simulink subsystem "control_filter"  (R2022b)
settings: Solver=VariableStepAuto  StartTime=0.0  StopTime=10.0  RelTol=1e-3
libraries: simulink x4, SG_library x1, hdlsllib x1
settings Model: Creator=mavolery  LastModifiedBy=mavolery

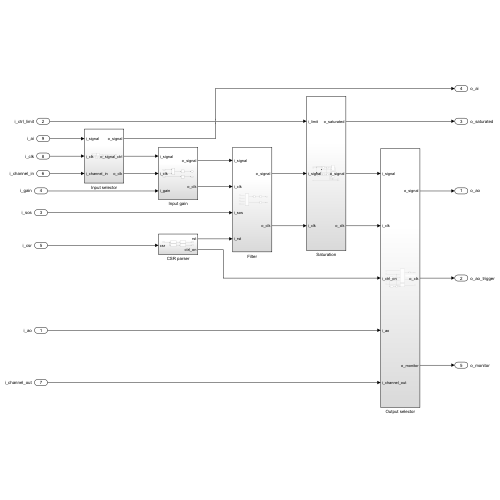
[thumbnail: Simulink's stored preview of the top-level diagram]
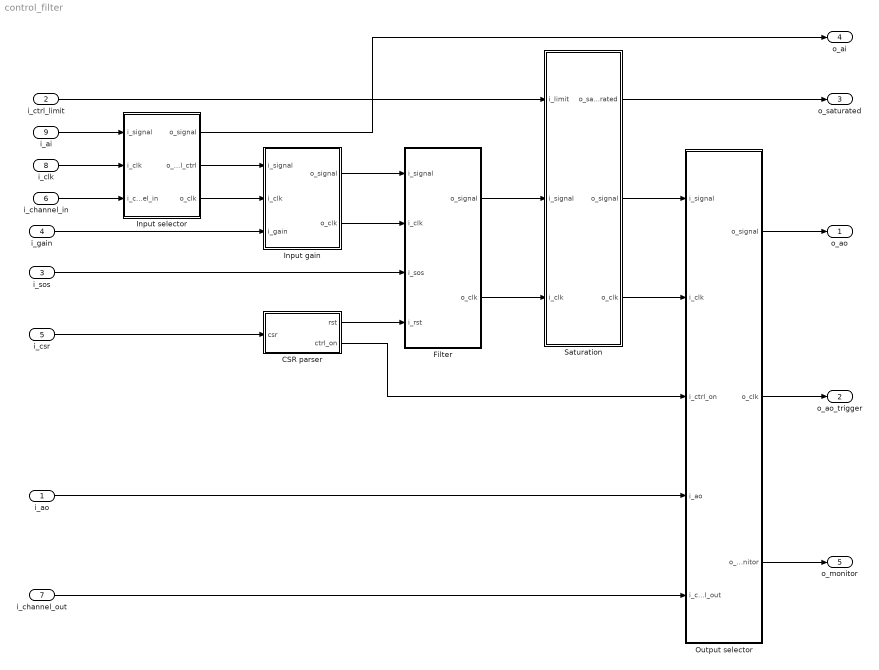
== system control_filter ==
  i_ao : Inport  OutDataTypeStr=fixdt(1,16,15)
  i_ctrl_limit : Inport  Port=2  OutDataTypeStr=fixdt(1,16,15)
  i_sos : Inport  Port=3  OutDataTypeStr=fixdt(1,32,26)
  i_gain : Inport  Port=4  OutDataTypeStr=fixdt(1,32,16)
  i_csr : Inport  Port=5  OutDataTypeStr=uint8
  i_channel_in : Inport  Port=6  OutDataTypeStr=uint8  PortDimensions=2
  i_channel_out : Inport  Port=7  OutDataTypeStr=uint8  PortDimensions=1
  i_clk : Inport  Port=8  OutDataTypeStr=boolean
  i_ai : Inport  Port=9  OutDataTypeStr=fixdt(1,16,15)
  CSR parser : Subsystem
  Filter : Subsystem
  Input gain : Subsystem
  Input selector : Subsystem
  Output selector : Subsystem
  Saturation : Subsystem
  o_ao : Outport  VectorParamsAs1DForOutWhenUnconnected=off
  o_ao_trigger : Outport  Port=2  VectorParamsAs1DForOutWhenUnconnected=off
  o_saturated : Outport  Port=3
  o_ai : Outport  Port=4
  o_monitor : Outport  Port=5
  wires:
  CSR parser/1(rst) -> Filter/4(i_rst)
  CSR parser/2(ctrl_on) -> Output selector/3(i_ctrl_on)
  i_ctrl_limit/1 -> Saturation/1(i_limit)
  i_csr/1 -> CSR parser/1(csr)
  Output selector/2(o_clk) -> o_ao_trigger/1
  Output selector/1(o_signal) -> o_ao/1
  i_sos/1 -> Filter/3(i_sos)
  i_ao/1 -> Output selector/4(i_ao)
  Input gain/1(o_signal) -> Filter/1(i_signal)
  Input gain/2(o_clk) -> Filter/2(i_clk)
  i_gain/1 -> Input gain/3(i_gain)
  i_ai/1 -> Input selector/1(i_signal)
  i_clk/1 -> Input selector/2(i_clk)
  Input selector/1(o_signal) -> o_ai/1
  Input selector/2(o_signal_ctrl) -> Input gain/1(i_signal)
  Input selector/3(o_clk) -> Input gain/2(i_clk)
  Filter/1(o_signal) -> Saturation/2(i_signal)
  Saturation/2(o_signal) -> Output selector/1(i_signal)
  Saturation/1(o_saturated) -> o_saturated/1
  Saturation/3(o_clk) -> Output selector/2(i_clk)
  Filter/2(o_clk) -> Saturation/3(i_clk)
  i_channel_in/1 -> Input selector/3(i_channel_in)
  i_channel_out/1 -> Output selector/5(i_channel_out)
  Output selector/3(o_monitor) -> o_monitor/1

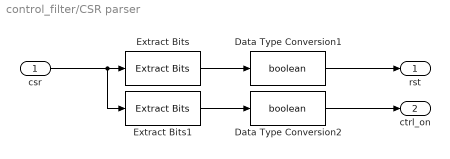
== system control_filter/CSR parser ==
  csr : Inport
  Data Type Conversion1 : DataTypeConversion  OutDataTypeStr=boolean  SaturateOnIntegerOverflow=off  RndMeth=Floor
  Data Type Conversion2 : DataTypeConversion  OutDataTypeStr=boolean  SaturateOnIntegerOverflow=off  RndMeth=Floor
  Extract Bits : simulink/Logic and Bit Operations/Extract Bits  bitsToExtract=Range of bits  numBits=8  bitIdxRange=0  outScalingMode=Treat bit field as an integer
  Extract Bits1 : simulink/Logic and Bit Operations/Extract Bits  bitsToExtract=Range of bits  numBits=8  bitIdxRange=1  outScalingMode=Treat bit field as an integer
  rst : Outport
  ctrl_on : Outport  Port=2
  wires:
  Extract Bits1/1 -> Data Type Conversion2/1
  csr/1 -> Extract Bits/1, Extract Bits1/1
  Data Type Conversion1/1 -> rst/1
  Extract Bits/1 -> Data Type Conversion1/1
  Data Type Conversion2/1 -> ctrl_on/1

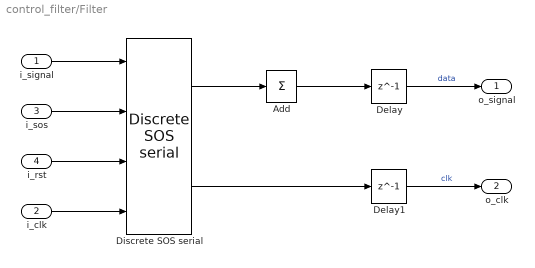
== system control_filter/Filter ==
  i_signal : Inport
  i_clk : Inport  Port=2
  i_sos : Inport  Port=3
  i_rst : Inport  Port=4
  Add : Sum  Inputs=+  SaturateOnIntegerOverflow=on  OutDataTypeStr=Inherit: Same as first input
  Delay : Delay  DelayLength=1
  Delay1 : Delay  DelayLength=1
  Discrete SOS serial : SG_library/Source elements/Discrete SOS serial  OutDataTypeStr=fixdt(1,80,52)
      settings: SourceProductName=Custom Speedgoat implementations
      settings: LibrarySourceBlock=|
      | SG_library/Source elements/Discrete SOS
      | serial DF1
  o_signal : Outport
  o_clk : Outport  Port=2
  wires:
  Delay1/1 -> o_clk/1  "clk"
  Delay/1 -> o_signal/1  "data"
  i_clk/1 -> Discrete SOS serial/4
  Discrete SOS serial/2 -> Delay1/1
  Add/1 -> Delay/1
  i_signal/1 -> Discrete SOS serial/1
  i_sos/1 -> Discrete SOS serial/2
  Discrete SOS serial/1 -> Add/1
  i_rst/1 -> Discrete SOS serial/3

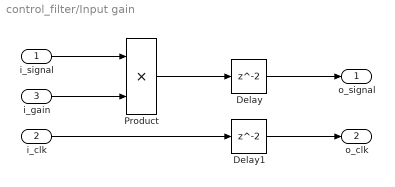
== system control_filter/Input gain ==
  i_signal : Inport
  i_clk : Inport  Port=2
  i_gain : Inport  Port=3
  Delay : Delay
  Delay1 : Delay
  Product : Product  OutDataTypeStr=Inherit: Same as first input
  o_signal : Outport
  o_clk : Outport  Port=2
  wires:
  i_clk/1 -> Delay1/1
  Delay1/1 -> o_clk/1
  Product/1 -> Delay/1
  Delay/1 -> o_signal/1
  i_gain/1 -> Product/2
  i_signal/1 -> Product/1

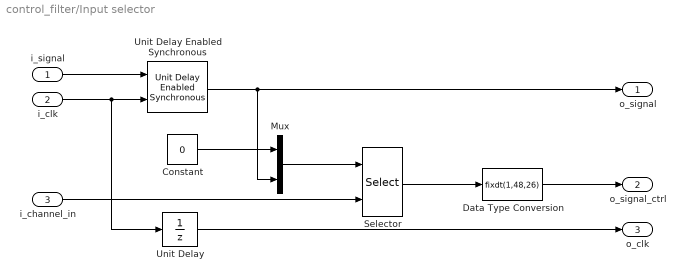
== system control_filter/Input selector ==
  i_signal : Inport
  i_clk : Inport  Port=2
  i_channel_in : Inport  Port=3  OutDataTypeStr=uint8  PortDimensions=2
  Constant : Constant  Value=0  OutDataTypeStr=Inherit: Inherit via back propagation  SampleTime=-1
  Data Type Conversion : DataTypeConversion  OutDataTypeStr=fixdt(1,48,26)  SaturateOnIntegerOverflow=off  RndMeth=Floor
  Mux : Mux  Inputs=2
  Selector : Selector  IndexMode=Zero-based  IndexOptions=Index vector (port)  Indices=1:2  OutputSizes=1
  Unit Delay : UnitDelay  SampleTime=-1  HasFrameUpgradeWarning=on
  Unit Delay Enabled Synchronous : hdlsllib/Discrete/Unit Delay Enabled Synchronous  InitialCondition=0.0  SampleTime=-1
  o_signal : Outport
  o_signal_ctrl : Outport  Port=2
  o_clk : Outport  Port=3
  wires:
  Constant/1 -> Mux/1
  Mux/1 -> Selector/1
  Unit Delay/1 -> o_clk/1
  Data Type Conversion/1 -> o_signal_ctrl/1
  Selector/1 -> Data Type Conversion/1
  Unit Delay Enabled Synchronous/1 -> o_signal/1, Mux/2
  i_clk/1 -> Unit Delay Enabled Synchronous/2, Unit Delay/1
  i_signal/1 -> Unit Delay Enabled Synchronous/1
  i_channel_in/1 -> Selector/2

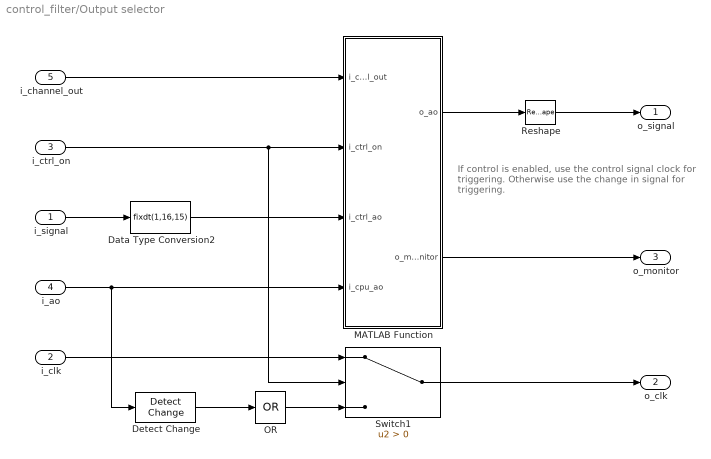
== system control_filter/Output selector ==
  note: If control is enabled, use the control signal clock for triggering. Otherwise use the change in signal for triggering.
  i_signal : Inport
  i_clk : Inport  Port=2
  i_ctrl_on : Inport  Port=3
  i_ao : Inport  Port=4
  i_channel_out : Inport  Port=5  OutDataTypeStr=uint8  PortDimensions=1
  Data Type Conversion2 : DataTypeConversion  OutDataTypeStr=fixdt(1,16,15)  RndMeth=Simplest
  Detect Change : simulink/Logic and Bit Operations/Detect Change  vinit=0  OutDataTypeStr=boolean
  MATLAB Function : MATLAB Function  TreatAsAtomicUnit=on
  OR : Logic  Operator=OR  Inputs=1  AllPortsSameDT=off  OutDataTypeStr=boolean
  Reshape : Reshape
  Switch1 : Switch  Criteria=u2 > Threshold  SaturateOnIntegerOverflow=off  InputSameDT=off
  o_signal : Outport
  o_clk : Outport  Port=2
  o_monitor : Outport  Port=3
  wires:
  i_ctrl_on/1 -> Switch1/2, MATLAB Function/2(i_ctrl_on)
  Detect Change/1 -> OR/1
  OR/1 -> Switch1/3
  Data Type Conversion2/1 -> MATLAB Function/3(i_ctrl_ao)
  Reshape/1 -> o_signal/1
  Switch1/1 -> o_clk/1
  i_ao/1 -> Detect Change/1, MATLAB Function/4(i_cpu_ao)
  MATLAB Function/1(o_ao) -> Reshape/1
  i_signal/1 -> Data Type Conversion2/1
  i_clk/1 -> Switch1/1
  i_channel_out/1 -> MATLAB Function/1(i_channel_out)
  MATLAB Function/2(o_monitor) -> o_monitor/1

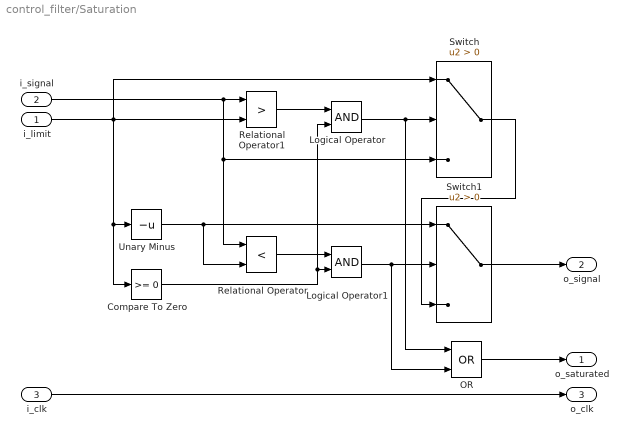
== system control_filter/Saturation ==
  i_limit : Inport
  i_signal : Inport  Port=2
  i_clk : Inport  Port=3
  Compare To Zero : simulink/Logic and Bit Operations/Compare To Zero  relop=>=  OutDataTypeStr=boolean
  Logical Operator : Logic  AllPortsSameDT=off  OutDataTypeStr=boolean
  Logical Operator1 : Logic  AllPortsSameDT=off  OutDataTypeStr=boolean
  OR : Logic  Operator=OR  AllPortsSameDT=off  OutDataTypeStr=boolean
  Relational Operator : RelationalOperator  Operator=<  OutDataTypeStr=boolean  RndMeth=Simplest  InputSameDT=off
  Relational Operator1 : RelationalOperator  Operator=>  OutDataTypeStr=boolean  RndMeth=Simplest  InputSameDT=off
  Switch : Switch  Criteria=u2 > Threshold  SaturateOnIntegerOverflow=off  InputSameDT=off
  Switch1 : Switch  Criteria=u2 > Threshold  SaturateOnIntegerOverflow=off  InputSameDT=off
  Unary Minus : UnaryMinus  SaturateOnIntegerOverflow=on
  o_saturated : Outport
  o_signal : Outport  Port=2
  o_clk : Outport  Port=3
  wires:
  i_clk/1 -> o_clk/1
  Logical Operator/1 -> OR/1, Switch/2
  Logical Operator1/1 -> OR/2, Switch1/2
  Compare To Zero/1 -> Logical Operator/2, Logical Operator1/2
  Relational Operator1/1 -> Logical Operator/1
  Relational Operator/1 -> Logical Operator1/1
  OR/1 -> o_saturated/1
  Switch1/1 -> o_signal/1
  Switch/1 -> Switch1/3
  i_signal/1 -> Switch/3, Relational Operator/1, Relational Operator1/1
  i_limit/1 -> Relational Operator1/2, Unary Minus/1, Compare To Zero/1, Switch/1
  Unary Minus/1 -> Relational Operator/2, Switch1/1

== matlab function control_filter/Output selector/MATLAB Function ==
  settings: fimath=fimath('RoundingMethod', 'Floor','OverflowAction', 'Wrap','ProductMode', 'FullPrecision', 'SumMode', 'FullPrecision')
  data: i_channel_out input; i_ctrl_on input; i_ctrl_ao input; i_cpu_ao input; o_ao output; o_monitor output
function [o_ao, o_monitor] = split(i_channel_out, i_ctrl_on, i_ctrl_ao, i_cpu_ao)
    o_ao = i_cpu_ao;
    o_monitor = zeros(size(i_ctrl_ao), 'like', i_ctrl_ao);
    if i_ctrl_on
        o_ao(i_channel_out) = i_ctrl_ao;
        o_monitor = i_ctrl_ao;
    end
end
